simulink model "Solution_01"  (R2018b)
settings: Solver=VariableStepAuto  StartTime=0.0  StopTime=10.0  RelTol=1e-3
settings Model: Creator=Gowtham  LastModifiedBy=Gowtham

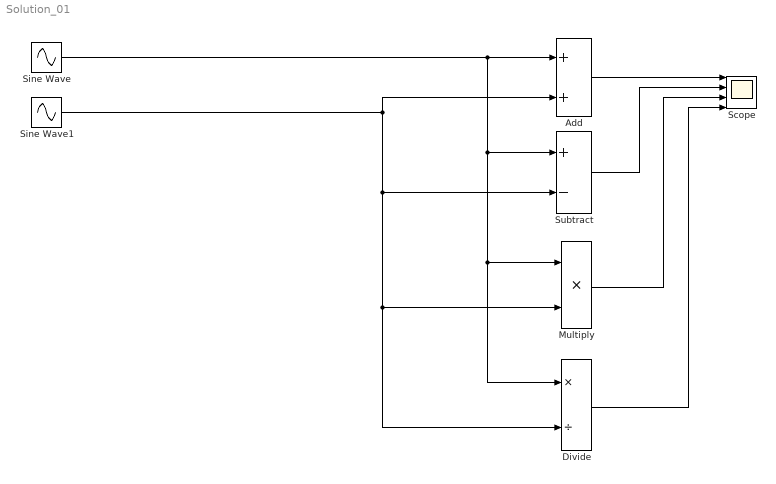
== system Solution_01 ==
  Add : Sum
  Divide : Product  Inputs=*/
  Multiply : Product
  Scope : Scope  NumInputPorts=4
  Sine Wave : Sin  SampleTime=0
  Sine Wave1 : Sin  SampleTime=0
  Subtract : Sum  Inputs=+-
  wires:
  Sine Wave/1 -> Multiply/1, Divide/1, Subtract/1, Add/1
  Sine Wave1/1 -> Add/2, Divide/2, Multiply/2, Subtract/2
  Add/1 -> Scope/1
  Subtract/1 -> Scope/2
  Multiply/1 -> Scope/3
  Divide/1 -> Scope/4
